simulink subsystem "Controller"  (R2025a)
settings: Solver=VariableStepAuto  StartTime=0.0  StopTime=10.0  RelTol=1e-3
undefined symbols (not defined in the file): config
settings Model: Creator=Jackt  LastModifiedBy=Jackt

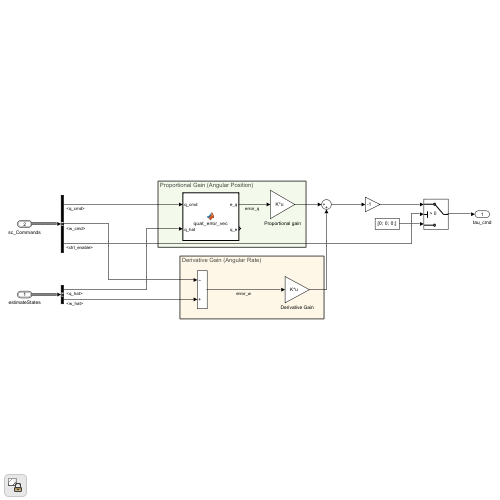
[thumbnail: Simulink's stored preview of the top-level diagram]
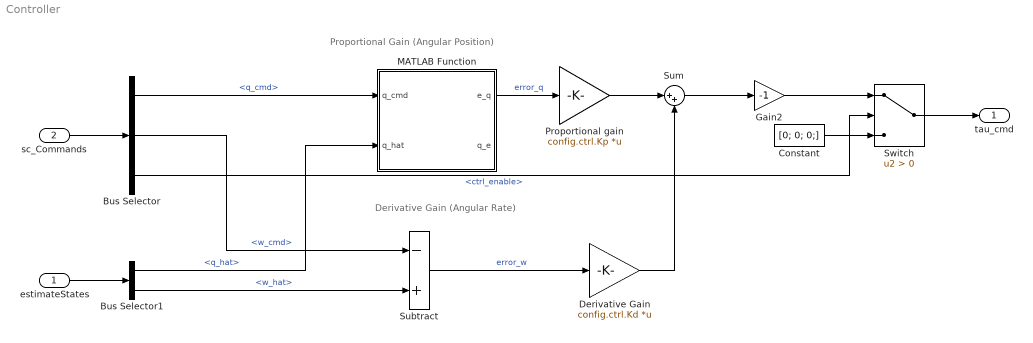
== system Controller ==
  note: Derivative Gain (Angular Rate)
  note: Proportional Gain (Angular Position)
  estimateStates : Inport  OutDataTypeStr=Bus: estimatedStateBus
  sc_Commands : Inport  Port=2  OutDataTypeStr=Bus: commandBus
  Bus Selector : BusSelector  OutputSignals=q_cmd,w_cmd,ctrl_enable
  Bus Selector1 : BusSelector  OutputSignals=q_hat,w_hat
  Constant : Constant  Value=[0; 0; 0;]
  Derivative Gain : Gain  Gain=config.ctrl.Kd  Multiplication=Matrix(K*u)
  Gain2 : Gain  Gain=-1
  MATLAB Function : MATLAB Function  TreatAsAtomicUnit=on
  Proportional gain : Gain  Gain=config.ctrl.Kp  Multiplication=Matrix(K*u)
  Subtract : Sum  Inputs=-+
  Sum : Sum  Inputs=|++
  Switch : Switch  Criteria=u2 > Threshold  SaturateOnIntegerOverflow=off  InputSameDT=off
  tau_cmd : Outport
  wires:
  Bus Selector/1 -> MATLAB Function/1(q_cmd)  "<q_cmd>"
  Bus Selector1/1 -> MATLAB Function/2(q_hat)  "<q_hat>"
  Bus Selector1/2 -> Subtract/2  "<w_hat>"
  Bus Selector/2 -> Subtract/1  "<w_cmd>"
  MATLAB Function/1(e_q) -> Proportional gain/1  "error_q"
  Subtract/1 -> Derivative Gain/1  "error_w"
  Proportional gain/1 -> Sum/1
  Sum/1 -> Gain2/1
  Derivative Gain/1 -> Sum/2
  Bus Selector/3 -> Switch/2  "<ctrl_enable>"
  Constant/1 -> Switch/3
  Switch/1 -> tau_cmd/1
  Gain2/1 -> Switch/1
  sc_Commands/1 -> Bus Selector/1
  estimateStates/1 -> Bus Selector1/1

== matlab function Controller/MATLAB Function ==
  data: q_cmd input; e_q output; q_hat input; q_e output
function [e_q, q_e] = quat_error_vec(q_cmd, q_hat)
%Calculate quaternion inverse (assume scalar first)
q_star = [q_cmd(1); -q_cmd(2); -q_cmd(3); -q_cmd(4)];
q_cmd_inv = q_star / norm(q_star)^2;

%Calculate q_e via hamilton product
q_e = quat_mul(q_cmd_inv, q_hat);

%Force quaternion to take the shortest route
if(q_e(1) < 0)
    q_e = -q_e;
end

%Convert to axis angle with log-mapping
s = q_e(1); %Scalar part
v = q_e(2:4); %Vector part
r = norm(v);

theta = 2 * atan2(r, s);

eps_r = 1e-9; %Machine precision
if(r < eps_r)
    e_q = [0; 0; 0];
else %If near machine precision
    e_q = theta * (v/r);
end

end

function q = quat_mul(p, r)
% p ⊗ r, both scalar-first
p0 = p(1); pv = p(2:4);
r0 = r(1); rv = r(2:4);

q0 = p0*r0 - dot(pv, rv);
qv = p0*rv + r0*pv + cross(pv, rv);

q = [q0; qv];
end
